simulink model "A3c"  (R2024a)
settings: Solver=ode45  StartTime=0  StopTime=15  MaxStep=0.01  RelTol=1e-3
libraries: simulink x1
settings Model: Creator=Flipper  LastModifiedBy=Flipper

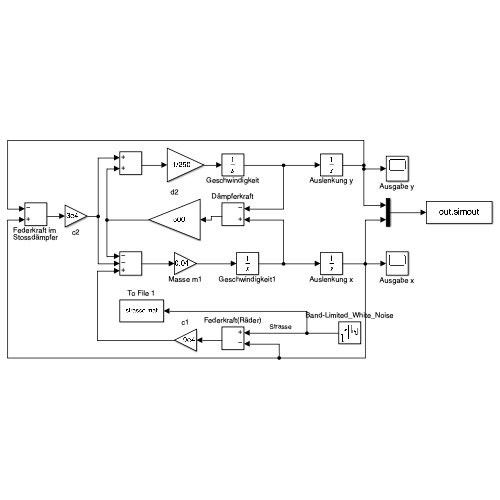
[thumbnail: Simulink's stored preview of the top-level diagram]
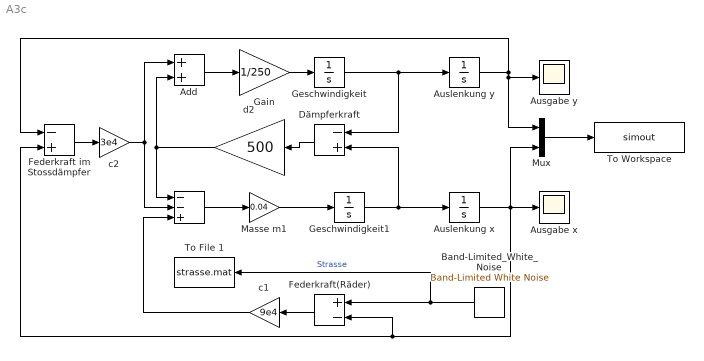
== system A3c ==
  " " : Sum  Inputs=--+
  Add : Sum
  Ausgabe x : Scope
  Ausgabe y : Scope
  Auslenkung x : Integrator
  Auslenkung y : Integrator
  Band-Limited_White_Noise : simulink/Sources/Band-Limited White Noise  Cov=0.0001  Ts=(2*pi)/(100*70)  seed=[23341]
  Dämpferkraft : Sum  Inputs=-+
  Federkraft im Stossdämpfer : Sum  Inputs=-+
  Federkraft(Räder) : Sum  Inputs=+-
  Gain : Gain  Gain=1/250
  Geschwindigkeit : Integrator
  Geschwindigkeit1 : Integrator
  Masse m1 : Gain  Gain=0.04
  Mux : Mux  Inputs=2
  To File 1 : ToFile  Filename=strasse.mat  SaveFormat=Timeseries
  To Workspace : ToWorkspace  VariableName=simout  SaveFormat=Timeseries  SampleTime=-1
  c1 : Gain  Gain=9e4
  c2 : Gain  Gain=3e4
  d2 : Gain  Gain=500
  wires:
  c2/1 -> " "/2, Add/1
  Gain/1 -> Geschwindigkeit/1
  Dämpferkraft/1 -> d2/1
  Auslenkung x/1 -> Federkraft im Stossdämpfer/2, Federkraft(Räder)/2, Ausgabe x/1, Mux/2
  Federkraft im Stossdämpfer/1 -> c2/1
  Mux/1 -> To Workspace/1
  d2/1 -> Add/2, " "/1
  Add/1 -> Gain/1
  Geschwindigkeit/1 -> Dämpferkraft/1, Auslenkung y/1
  Geschwindigkeit1/1 -> Auslenkung x/1, Dämpferkraft/2
  Masse m1/1 -> Geschwindigkeit1/1
  " "/1 -> Masse m1/1
  Federkraft(Räder)/1 -> c1/1
  Auslenkung y/1 -> Mux/1, Ausgabe y/1, Federkraft im Stossdämpfer/1
  c1/1 -> " "/3
  Band-Limited_White_Noise/1 -> To File 1/1, Federkraft(Räder)/1  "Strasse"
